simulink library "relay_housing_lib"  (Simulink 8.1)
settings: Solver=ode45  StartTime=0.0  StopTime=10.0  RelTol=1e-3
values from neighbouring files (symbols this model uses):
  F1 = xlsread('F1_relay_banshee.xlsx')    [relay_settings_init.m]
  F2 = xlsread('F2_relay_banshee.xlsx')    [relay_settings_init.m]
  F3 = xlsread('F3_relay_banshee.xlsx')    [relay_settings_init.m]
  Ts = 100E-6    (= 0.0001)    [BANSHEE_init.m]
libraries: relay_modbus_lib x42, rtio_generic_modbus x42, rtlab x3, LoadProfiles_lib x1
settings Model: Creator=re25624  LastModifiedBy=re25624

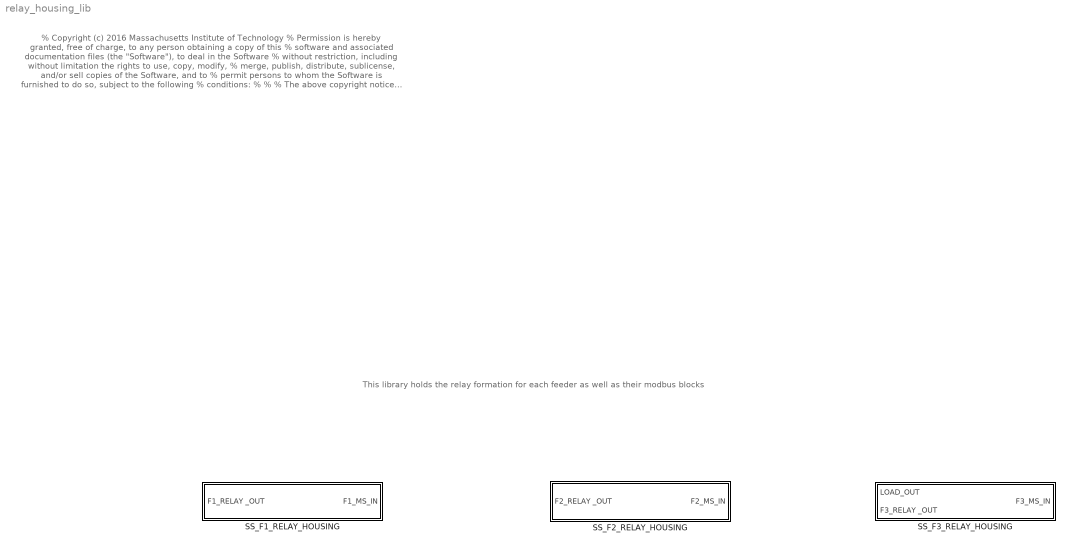
== system relay_housing_lib ==
  note: This library holds the relay formation for each feeder as well as their modbus blocks
  note: % Copyright (c) 2016 Massachusetts Institute of Technology
      | % Permission is hereby granted, free of charge, to any person obtaining a copy of this
      | % software and associated documentation files (the "Software"), to deal in the Software
      | % without restriction, including without limitation the rights to use, copy, modify,
      | % merge, publish, distribute, sublicense, and/or sell copies of the Software, and to
      | % permit persons to whom the Software is furnished to do so, subject to the following
      | % conditions:
      | %
      | %
      | % The above copyright notice and this permission notice shall be included in
      | % all copies or substantial portions of the Software.
      | %
      | % THE SOFTWARE IS PROVIDED "AS IS", WITHOUT WARRANTY OF ANY KIND, EXPRESS OR IMPLIED,
      | % INCLUDING BUT NOT LIMITED TO THE WARRANTIES OF MERCHANTABILITY, FITNESS FOR A
      | % PARTICULAR PURPOSE AND NONINFRINGEMENT. IN NO EVENT SHALL THE AUTHORS OR COPYRIGHT
      | % HOLDERS BE LIABLE FOR ANY CLAIM, DAMAGES OR OTHER LIABILITY, WHETHER IN AN ACTION
      | % OF CONTRACT, TORT OR OTHERWISE, ARISING FROM, OUT OF OR IN CONNECTION WITH THE
      | % SOFTWARE OR THE USE OR OTHER DEALINGS IN THE SOFTWARE.
      | %
      | %
      | %%
  SS_F1_RELAY_HOUSING : Subsystem
  SS_F2_RELAY_HOUSING : Subsystem
  SS_F3_RELAY_HOUSING : Subsystem

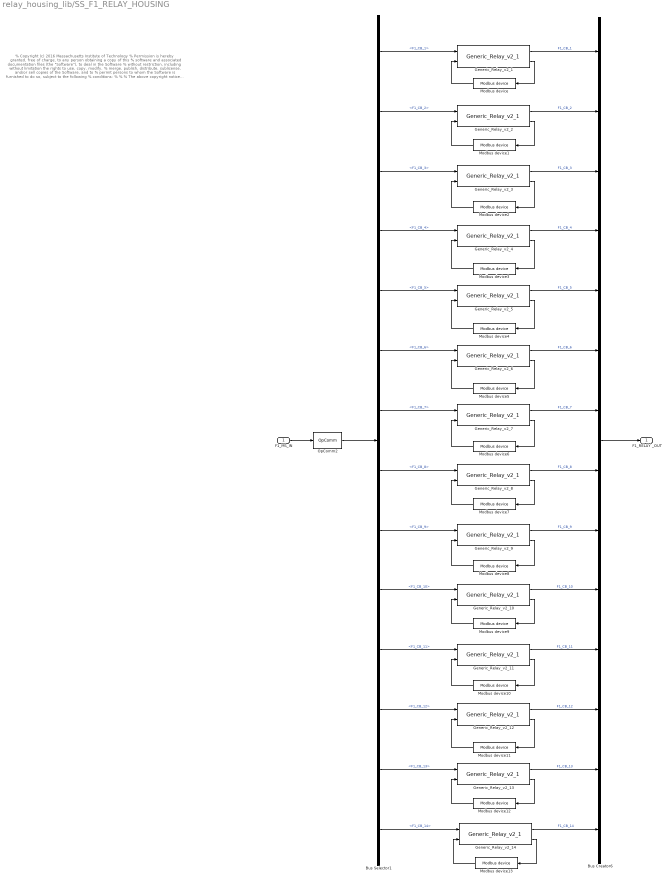
== system relay_housing_lib/SS_F1_RELAY_HOUSING ==
  note: % Copyright (c) 2016 Massachusetts Institute of Technology
      | % Permission is hereby granted, free of charge, to any person obtaining a copy of this
      | % software and associated documentation files (the "Software"), to deal in the Software
      | % without restriction, including without limitation the rights to use, copy, modify,
      | % merge, publish, distribute, sublicense, and/or sell copies of the Software, and to
      | % permit persons to whom the Software is furnished to do so, subject to the following
      | % conditions:
      | %
      | %
      | % The above copyright notice and this permission notice shall be included in
      | % all copies or substantial portions of the Software.
      | %
      | % THE SOFTWARE IS PROVIDED "AS IS", WITHOUT WARRANTY OF ANY KIND, EXPRESS OR IMPLIED,
      | % INCLUDING BUT NOT LIMITED TO THE WARRANTIES OF MERCHANTABILITY, FITNESS FOR A
      | % PARTICULAR PURPOSE AND NONINFRINGEMENT. IN NO EVENT SHALL THE AUTHORS OR COPYRIGHT
      | % HOLDERS BE LIABLE FOR ANY CLAIM, DAMAGES OR OTHER LIABILITY, WHETHER IN AN ACTION
      | % OF CONTRACT, TORT OR OTHERWISE, ARISING FROM, OUT OF OR IN CONNECTION WITH THE
      | % SOFTWARE OR THE USE OR OTHER DEALINGS IN THE SOFTWARE.
      | %
      | %
      | %%
  F1_MS_IN : Inport
  Bus Creator6 : BusCreator  Inputs=14
  Bus Selector1 : BusSelector  OutputSignals=F1_CB_1,F1_CB_2,F1_CB_3,F1_CB_4,F1_CB_5,F1_CB_6,F1_CB_7,F1_CB_8,F1_CB_9,F1_CB_10,F1_CB_11,F1_CB_12,F1_CB_13,F1_CB_14
  Generic_Relay_v2_1 : relay_modbus_lib/Generic_Relay_v2_1  Ts=Ts  relay_settings=[F1(1,:)]
  Generic_Relay_v2_10 : relay_modbus_lib/Generic_Relay_v2_1  Ts=Ts  relay_settings=[F1(10,:)]
  Generic_Relay_v2_11 : relay_modbus_lib/Generic_Relay_v2_1  Ts=Ts  relay_settings=[F1(11,:)]
  Generic_Relay_v2_12 : relay_modbus_lib/Generic_Relay_v2_1  Ts=Ts  relay_settings=[F1(12,:)]
  Generic_Relay_v2_13 : relay_modbus_lib/Generic_Relay_v2_1  Ts=Ts  relay_settings=[F1(13,:)]
  Generic_Relay_v2_14 : relay_modbus_lib/Generic_Relay_v2_1  Ts=Ts  relay_settings=[F1(14,:)]
  Generic_Relay_v2_2 : relay_modbus_lib/Generic_Relay_v2_1  Ts=Ts  relay_settings=[F1(2,:)]
  Generic_Relay_v2_3 : relay_modbus_lib/Generic_Relay_v2_1  Ts=Ts  relay_settings=[F1(3,:)]
  Generic_Relay_v2_4 : relay_modbus_lib/Generic_Relay_v2_1  Ts=Ts  relay_settings=[F1(4,:)]
  Generic_Relay_v2_5 : relay_modbus_lib/Generic_Relay_v2_1  Ts=Ts  relay_settings=[F1(5,:)]
  Generic_Relay_v2_6 : relay_modbus_lib/Generic_Relay_v2_1  Ts=Ts  relay_settings=[F1(6,:)]
  Generic_Relay_v2_7 : relay_modbus_lib/Generic_Relay_v2_1  Ts=Ts  relay_settings=[F1(7,:)]
  Generic_Relay_v2_8 : relay_modbus_lib/Generic_Relay_v2_1  Ts=Ts  relay_settings=[F1(8,:)]
  Generic_Relay_v2_9 : relay_modbus_lib/Generic_Relay_v2_1  Ts=Ts  relay_settings=[F1(9,:)]
  Modbus device : rtio_generic_modbus/Modbus device  conf_name=F1_relay_cfg1.opal  conf_name_mask=F1_relay_cfg1.xls  sample_time=Ts
  Modbus device1 : rtio_generic_modbus/Modbus device  conf_name=F1_relay_cfg2.opal  conf_name_mask=F1_relay_cfg2.xls  sample_time=Ts
  Modbus device10 : rtio_generic_modbus/Modbus device  conf_name=F1_relay_cfg11.opal  conf_name_mask=F1_relay_cfg11.xls  sample_time=Ts
  Modbus device11 : rtio_generic_modbus/Modbus device  conf_name=F1_relay_cfg12.opal  conf_name_mask=F1_relay_cfg12.xls  sample_time=Ts
  Modbus device12 : rtio_generic_modbus/Modbus device  conf_name=F1_relay_cfg13.opal  conf_name_mask=F1_relay_cfg13.xls  sample_time=Ts
  Modbus device13 : rtio_generic_modbus/Modbus device  conf_name=F1_relay_cfg14.opal  conf_name_mask=F1_relay_cfg14.xls  sample_time=Ts
  Modbus device2 : rtio_generic_modbus/Modbus device  conf_name=F1_relay_cfg3.opal  conf_name_mask=F1_relay_cfg3.xls  sample_time=Ts
  Modbus device3 : rtio_generic_modbus/Modbus device  conf_name=F1_relay_cfg4.opal  conf_name_mask=F1_relay_cfg4.xls  sample_time=Ts
  Modbus device4 : rtio_generic_modbus/Modbus device  conf_name=F1_relay_cfg5.opal  conf_name_mask=F1_relay_cfg5.xls  sample_time=Ts
  Modbus device5 : rtio_generic_modbus/Modbus device  conf_name=F1_relay_cfg6.opal  conf_name_mask=F1_relay_cfg6.xls  sample_time=Ts
  Modbus device6 : rtio_generic_modbus/Modbus device  conf_name=F1_relay_cfg7.opal  conf_name_mask=F1_relay_cfg7.xls  sample_time=Ts
  Modbus device7 : rtio_generic_modbus/Modbus device  conf_name=F1_relay_cfg8.opal  conf_name_mask=F1_relay_cfg8.xls  sample_time=Ts
  Modbus device8 : rtio_generic_modbus/Modbus device  conf_name=F1_relay_cfg9.opal  conf_name_mask=F1_relay_cfg9.xls  sample_time=Ts
  Modbus device9 : rtio_generic_modbus/Modbus device  conf_name=F1_relay_cfg10.opal  conf_name_mask=F1_relay_cfg10.xls  sample_time=Ts
  OpComm2 : rtlab/OpComm  nbport=1  groupe_acq=1  subsys_rate=0  st=0  Synchronization=on  Interpolation=on  Threshold=1.0  Missed_Data=off  Sim_Time=off  Samples=off  dynSigOut=off  from_console=0  warning_done=off  writeOpCommFile=off  Offset=off
  F1_RELAY _OUT : Outport
  wires:
  Bus Selector1/14 -> Generic_Relay_v2_14/1  "<F1_CB_14>"
  Generic_Relay_v2_14/1 -> Bus Creator6/14  "F1_CB_14"
  Generic_Relay_v2_14/2 -> Modbus device13/1
  Modbus device13/1 -> Generic_Relay_v2_14/2
  Generic_Relay_v2_3/1 -> Bus Creator6/3  "F1_CB_3"
  Generic_Relay_v2_4/1 -> Bus Creator6/4  "F1_CB_4"
  Generic_Relay_v2_5/1 -> Bus Creator6/5  "F1_CB_5"
  Generic_Relay_v2_6/1 -> Bus Creator6/6  "F1_CB_6"
  Generic_Relay_v2_7/1 -> Bus Creator6/7  "F1_CB_7"
  Generic_Relay_v2_8/1 -> Bus Creator6/8  "F1_CB_8"
  Generic_Relay_v2_9/1 -> Bus Creator6/9  "F1_CB_9"
  Generic_Relay_v2_10/1 -> Bus Creator6/10  "F1_CB_10"
  Generic_Relay_v2_11/1 -> Bus Creator6/11  "F1_CB_11"
  Generic_Relay_v2_12/1 -> Bus Creator6/12  "F1_CB_12"
  Generic_Relay_v2_13/1 -> Bus Creator6/13  "F1_CB_13"
  Bus Selector1/13 -> Generic_Relay_v2_13/1  "<F1_CB_13>"
  Bus Selector1/12 -> Generic_Relay_v2_12/1  "<F1_CB_12>"
  Bus Selector1/11 -> Generic_Relay_v2_11/1  "<F1_CB_11>"
  Bus Selector1/10 -> Generic_Relay_v2_10/1  "<F1_CB_10>"
  Bus Selector1/9 -> Generic_Relay_v2_9/1  "<F1_CB_9>"
  Bus Selector1/8 -> Generic_Relay_v2_8/1  "<F1_CB_8>"
  Bus Selector1/7 -> Generic_Relay_v2_7/1  "<F1_CB_7>"
  Bus Selector1/6 -> Generic_Relay_v2_6/1  "<F1_CB_6>"
  Bus Selector1/5 -> Generic_Relay_v2_5/1  "<F1_CB_5>"
  Bus Selector1/4 -> Generic_Relay_v2_4/1  "<F1_CB_4>"
  Bus Selector1/3 -> Generic_Relay_v2_3/1  "<F1_CB_3>"
  Generic_Relay_v2_2/1 -> Bus Creator6/2  "F1_CB_2"
  Bus Selector1/2 -> Generic_Relay_v2_2/1  "<F1_CB_2>"
  Bus Creator6/1 -> F1_RELAY _OUT/1
  Generic_Relay_v2_1/1 -> Bus Creator6/1  "F1_CB_1"
  Bus Selector1/1 -> Generic_Relay_v2_1/1  "<F1_CB_1>"
  F1_MS_IN/1 -> OpComm2/1
  Modbus device/1 -> Generic_Relay_v2_1/2
  Generic_Relay_v2_1/2 -> Modbus device/1
  Modbus device1/1 -> Generic_Relay_v2_2/2
  Generic_Relay_v2_2/2 -> Modbus device1/1
  Generic_Relay_v2_3/2 -> Modbus device2/1
  Modbus device2/1 -> Generic_Relay_v2_3/2
  Generic_Relay_v2_4/2 -> Modbus device3/1
  Modbus device3/1 -> Generic_Relay_v2_4/2
  Generic_Relay_v2_5/2 -> Modbus device4/1
  Modbus device4/1 -> Generic_Relay_v2_5/2
  Generic_Relay_v2_6/2 -> Modbus device5/1
  Modbus device5/1 -> Generic_Relay_v2_6/2
  Generic_Relay_v2_7/2 -> Modbus device6/1
  Modbus device6/1 -> Generic_Relay_v2_7/2
  Generic_Relay_v2_8/2 -> Modbus device7/1
  Modbus device7/1 -> Generic_Relay_v2_8/2
  Generic_Relay_v2_9/2 -> Modbus device8/1
  Modbus device8/1 -> Generic_Relay_v2_9/2
  Generic_Relay_v2_10/2 -> Modbus device9/1
  Modbus device9/1 -> Generic_Relay_v2_10/2
  Generic_Relay_v2_11/2 -> Modbus device10/1
  Modbus device10/1 -> Generic_Relay_v2_11/2
  Generic_Relay_v2_12/2 -> Modbus device11/1
  Modbus device11/1 -> Generic_Relay_v2_12/2
  Generic_Relay_v2_13/2 -> Modbus device12/1
  Modbus device12/1 -> Generic_Relay_v2_13/2
  OpComm2/1 -> Bus Selector1/1

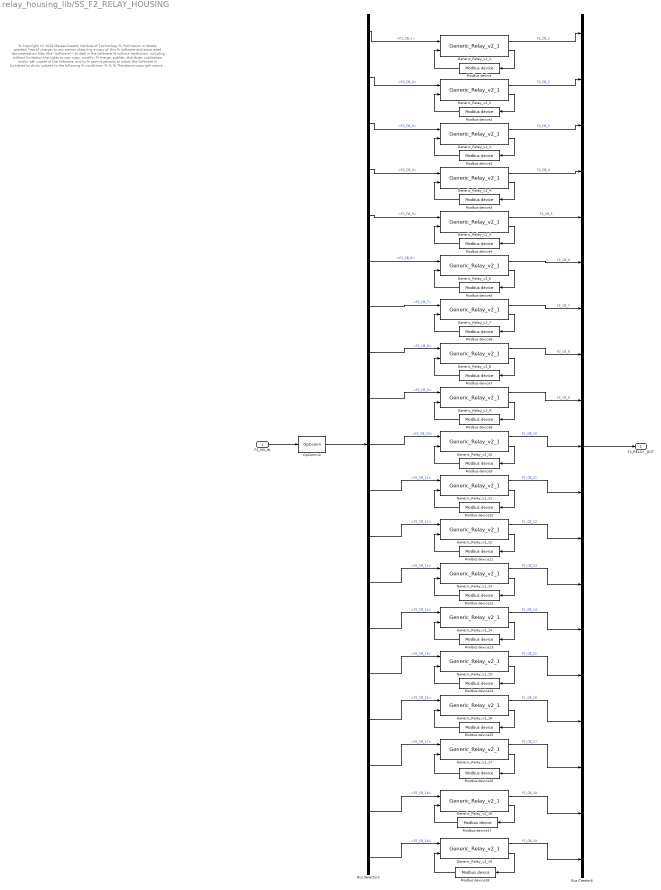
== system relay_housing_lib/SS_F2_RELAY_HOUSING ==
  note: % Copyright (c) 2016 Massachusetts Institute of Technology
      | % Permission is hereby granted, free of charge, to any person obtaining a copy of this
      | % software and associated documentation files (the "Software"), to deal in the Software
      | % without restriction, including without limitation the rights to use, copy, modify,
      | % merge, publish, distribute, sublicense, and/or sell copies of the Software, and to
      | % permit persons to whom the Software is furnished to do so, subject to the following
      | % conditions:
      | %
      | %
      | % The above copyright notice and this permission notice shall be included in
      | % all copies or substantial portions of the Software.
      | %
      | % THE SOFTWARE IS PROVIDED "AS IS", WITHOUT WARRANTY OF ANY KIND, EXPRESS OR IMPLIED,
      | % INCLUDING BUT NOT LIMITED TO THE WARRANTIES OF MERCHANTABILITY, FITNESS FOR A
      | % PARTICULAR PURPOSE AND NONINFRINGEMENT. IN NO EVENT SHALL THE AUTHORS OR COPYRIGHT
      | % HOLDERS BE LIABLE FOR ANY CLAIM, DAMAGES OR OTHER LIABILITY, WHETHER IN AN ACTION
      | % OF CONTRACT, TORT OR OTHERWISE, ARISING FROM, OUT OF OR IN CONNECTION WITH THE
      | % SOFTWARE OR THE USE OR OTHER DEALINGS IN THE SOFTWARE.
      | %
      | %
      | %%
  F2_MS_IN : Inport
  Bus Creator6 : BusCreator  Inputs=19
  Bus Selector2 : BusSelector  OutputSignals=F2_CB_1,F2_CB_2,F2_CB_3,F2_CB_4,F2_CB_5,F2_CB_6,F2_CB_7,F2_CB_8,F2_CB_9,F2_CB_10,F2_CB_11,F2_CB_12,F2_CB_13,F2_CB_14,F2_CB_15,F2_CB_16,F2_CB_17,F2_CB_18,F2_CB_19
  Generic_Relay_v2_1 : relay_modbus_lib/Generic_Relay_v2_1  Ts=Ts  relay_settings=[F2(1,:)]
  Generic_Relay_v2_10 : relay_modbus_lib/Generic_Relay_v2_1  Ts=Ts  relay_settings=[F2(10,:)]
  Generic_Relay_v2_11 : relay_modbus_lib/Generic_Relay_v2_1  Ts=Ts  relay_settings=[F2(11,:)]
  Generic_Relay_v2_12 : relay_modbus_lib/Generic_Relay_v2_1  Ts=Ts  relay_settings=[F2(12,:)]
  Generic_Relay_v2_13 : relay_modbus_lib/Generic_Relay_v2_1  Ts=Ts  relay_settings=[F2(13,:)]
  Generic_Relay_v2_14 : relay_modbus_lib/Generic_Relay_v2_1  Ts=Ts  relay_settings=[F2(14,:)]
  Generic_Relay_v2_15 : relay_modbus_lib/Generic_Relay_v2_1  Ts=Ts  relay_settings=[F2(15,:)]
  Generic_Relay_v2_16 : relay_modbus_lib/Generic_Relay_v2_1  Ts=Ts  relay_settings=[F2(16,:)]
  Generic_Relay_v2_17 : relay_modbus_lib/Generic_Relay_v2_1  Ts=Ts  relay_settings=[F2(17,:)]
  Generic_Relay_v2_18 : relay_modbus_lib/Generic_Relay_v2_1  Ts=Ts  relay_settings=[F2(18,:)]
  Generic_Relay_v2_19 : relay_modbus_lib/Generic_Relay_v2_1  Ts=Ts  relay_settings=[F2(19,:)]
  Generic_Relay_v2_2 : relay_modbus_lib/Generic_Relay_v2_1  Ts=Ts  relay_settings=[F2(2,:)]
  Generic_Relay_v2_3 : relay_modbus_lib/Generic_Relay_v2_1  Ts=Ts  relay_settings=[F2(3,:)]
  Generic_Relay_v2_4 : relay_modbus_lib/Generic_Relay_v2_1  Ts=Ts  relay_settings=[F2(4,:)]
  Generic_Relay_v2_5 : relay_modbus_lib/Generic_Relay_v2_1  Ts=Ts  relay_settings=[F2(5,:)]
  Generic_Relay_v2_6 : relay_modbus_lib/Generic_Relay_v2_1  Ts=Ts  relay_settings=[F2(6,:)]
  Generic_Relay_v2_7 : relay_modbus_lib/Generic_Relay_v2_1  Ts=Ts  relay_settings=[F2(7,:)]
  Generic_Relay_v2_8 : relay_modbus_lib/Generic_Relay_v2_1  Ts=Ts  relay_settings=[F2(8,:)]
  Generic_Relay_v2_9 : relay_modbus_lib/Generic_Relay_v2_1  Ts=Ts  relay_settings=[F2(9,:)]
  Modbus device : rtio_generic_modbus/Modbus device  conf_name=F2_relay_cfg1.opal  conf_name_mask=F2_relay_cfg1.xls  sample_time=Ts
  Modbus device1 : rtio_generic_modbus/Modbus device  conf_name=F2_relay_cfg2.opal  conf_name_mask=F2_relay_cfg2.xls  sample_time=Ts
  Modbus device10 : rtio_generic_modbus/Modbus device  conf_name=F2_relay_cfg11.opal  conf_name_mask=F2_relay_cfg11.xls  sample_time=Ts
  Modbus device11 : rtio_generic_modbus/Modbus device  conf_name=F2_relay_cfg12.opal  conf_name_mask=F2_relay_cfg12.xls  sample_time=Ts
  Modbus device12 : rtio_generic_modbus/Modbus device  conf_name=F2_relay_cfg13.opal  conf_name_mask=F2_relay_cfg13.xls  sample_time=Ts
  Modbus device13 : rtio_generic_modbus/Modbus device  conf_name=F2_relay_cfg14.opal  conf_name_mask=F2_relay_cfg14.xls  sample_time=Ts
  Modbus device14 : rtio_generic_modbus/Modbus device  conf_name=F2_relay_cfg15.opal  conf_name_mask=F2_relay_cfg15.xls  sample_time=Ts
  Modbus device15 : rtio_generic_modbus/Modbus device  conf_name=F2_relay_cfg16.opal  conf_name_mask=F2_relay_cfg16.xls  sample_time=Ts
  Modbus device16 : rtio_generic_modbus/Modbus device  conf_name=F2_relay_cfg17.opal  conf_name_mask=F2_relay_cfg17.xls  sample_time=Ts
  Modbus device17 : rtio_generic_modbus/Modbus device  conf_name=F2_relay_cfg18.opal  conf_name_mask=F2_relay_cfg18.xls  sample_time=Ts
  Modbus device18 : rtio_generic_modbus/Modbus device  conf_name=F2_relay_cfg19.opal  conf_name_mask=F2_relay_cfg19.xls  sample_time=Ts
  Modbus device2 : rtio_generic_modbus/Modbus device  conf_name=F2_relay_cfg3.opal  conf_name_mask=F2_relay_cfg3.xls  sample_time=Ts
  Modbus device3 : rtio_generic_modbus/Modbus device  conf_name=F2_relay_cfg4.opal  conf_name_mask=F2_relay_cfg4.xls  sample_time=Ts
  Modbus device4 : rtio_generic_modbus/Modbus device  conf_name=F2_relay_cfg5.opal  conf_name_mask=F2_relay_cfg5.xls  sample_time=Ts
  Modbus device5 : rtio_generic_modbus/Modbus device  conf_name=F2_relay_cfg6.opal  conf_name_mask=F2_relay_cfg6.xls  sample_time=Ts
  Modbus device6 : rtio_generic_modbus/Modbus device  conf_name=F2_relay_cfg7.opal  conf_name_mask=F2_relay_cfg7.xls  sample_time=Ts
  Modbus device7 : rtio_generic_modbus/Modbus device  conf_name=F2_relay_cfg8.opal  conf_name_mask=F2_relay_cfg8.xls  sample_time=Ts
  Modbus device8 : rtio_generic_modbus/Modbus device  conf_name=F2_relay_cfg9.opal  conf_name_mask=F2_relay_cfg9.xls  sample_time=Ts
  Modbus device9 : rtio_generic_modbus/Modbus device  conf_name=F2_relay_cfg10.opal  conf_name_mask=F2_relay_cfg10.xls  sample_time=Ts
  OpComm2 : rtlab/OpComm  nbport=1  groupe_acq=1  subsys_rate=0  st=0  Synchronization=on  Interpolation=on  Threshold=1.0  Missed_Data=off  Sim_Time=off  Samples=off  dynSigOut=off  from_console=0  warning_done=off  writeOpCommFile=off  Offset=off
  F2_RELAY _OUT : Outport
  wires:
  Bus Selector2/18 -> Generic_Relay_v2_18/1  "<F2_CB_18>"
  Bus Selector2/19 -> Generic_Relay_v2_19/1  "<F2_CB_19>"
  Generic_Relay_v2_19/1 -> Bus Creator6/19  "F2_CB_19"
  Generic_Relay_v2_18/1 -> Bus Creator6/18  "F2_CB_18"
  Generic_Relay_v2_18/2 -> Modbus device17/1
  Modbus device17/1 -> Generic_Relay_v2_18/2
  Generic_Relay_v2_19/2 -> Modbus device18/1
  Modbus device18/1 -> Generic_Relay_v2_19/2
  Bus Selector2/17 -> Generic_Relay_v2_17/1  "<F2_CB_17>"
  Generic_Relay_v2_17/1 -> Bus Creator6/17  "F2_CB_17"
  Generic_Relay_v2_6/1 -> Bus Creator6/6  "F2_CB_6"
  Generic_Relay_v2_5/1 -> Bus Creator6/5  "F2_CB_5"
  Generic_Relay_v2_4/1 -> Bus Creator6/4  "F2_CB_4"
  Generic_Relay_v2_3/1 -> Bus Creator6/3  "F2_CB_3"
  Generic_Relay_v2_2/1 -> Bus Creator6/2  "F2_CB_2"
  Generic_Relay_v2_7/1 -> Bus Creator6/7  "F2_CB_7"
  Generic_Relay_v2_8/1 -> Bus Creator6/8  "F2_CB_8"
  Generic_Relay_v2_9/1 -> Bus Creator6/9  "F2_CB_9"
  Generic_Relay_v2_10/1 -> Bus Creator6/10  "F2_CB_10"
  Generic_Relay_v2_11/1 -> Bus Creator6/11  "F2_CB_11"
  Generic_Relay_v2_16/1 -> Bus Creator6/16  "F2_CB_16"
  Generic_Relay_v2_15/1 -> Bus Creator6/15  "F2_CB_15"
  Generic_Relay_v2_14/1 -> Bus Creator6/14  "F2_CB_14"
  Generic_Relay_v2_13/1 -> Bus Creator6/13  "F2_CB_13"
  Generic_Relay_v2_12/1 -> Bus Creator6/12  "F2_CB_12"
  Bus Selector2/16 -> Generic_Relay_v2_16/1  "<F2_CB_16>"
  Bus Selector2/15 -> Generic_Relay_v2_15/1  "<F2_CB_15>"
  Bus Selector2/14 -> Generic_Relay_v2_14/1  "<F2_CB_14>"
  Bus Selector2/13 -> Generic_Relay_v2_13/1  "<F2_CB_13>"
  Bus Selector2/12 -> Generic_Relay_v2_12/1  "<F2_CB_12>"
  Bus Selector2/11 -> Generic_Relay_v2_11/1  "<F2_CB_11>"
  Bus Selector2/10 -> Generic_Relay_v2_10/1  "<F2_CB_10>"
  Bus Selector2/9 -> Generic_Relay_v2_9/1  "<F2_CB_9>"
  Bus Selector2/8 -> Generic_Relay_v2_8/1  "<F2_CB_8>"
  Bus Selector2/7 -> Generic_Relay_v2_7/1  "<F2_CB_7>"
  Bus Selector2/6 -> Generic_Relay_v2_6/1  "<F2_CB_6>"
  Bus Selector2/5 -> Generic_Relay_v2_5/1  "<F2_CB_5>"
  Bus Selector2/4 -> Generic_Relay_v2_4/1  "<F2_CB_4>"
  Bus Selector2/3 -> Generic_Relay_v2_3/1  "<F2_CB_3>"
  Bus Selector2/2 -> Generic_Relay_v2_2/1  "<F2_CB_2>"
  Generic_Relay_v2_1/1 -> Bus Creator6/1  "F2_CB_1"
  Bus Selector2/1 -> Generic_Relay_v2_1/1  "<F2_CB_1>"
  F2_MS_IN/1 -> OpComm2/1
  Bus Creator6/1 -> F2_RELAY _OUT/1
  Generic_Relay_v2_1/2 -> Modbus device/1
  Modbus device/1 -> Generic_Relay_v2_1/2
  Generic_Relay_v2_2/2 -> Modbus device1/1
  Modbus device1/1 -> Generic_Relay_v2_2/2
  Generic_Relay_v2_3/2 -> Modbus device2/1
  Modbus device2/1 -> Generic_Relay_v2_3/2
  Generic_Relay_v2_4/2 -> Modbus device3/1
  Modbus device3/1 -> Generic_Relay_v2_4/2
  Generic_Relay_v2_5/2 -> Modbus device4/1
  Modbus device4/1 -> Generic_Relay_v2_5/2
  Modbus device5/1 -> Generic_Relay_v2_6/2
  Generic_Relay_v2_6/2 -> Modbus device5/1
  Generic_Relay_v2_7/2 -> Modbus device6/1
  Modbus device6/1 -> Generic_Relay_v2_7/2
  Generic_Relay_v2_8/2 -> Modbus device7/1
  Modbus device7/1 -> Generic_Relay_v2_8/2
  Generic_Relay_v2_9/2 -> Modbus device8/1
  Modbus device8/1 -> Generic_Relay_v2_9/2
  Generic_Relay_v2_10/2 -> Modbus device9/1
  Modbus device9/1 -> Generic_Relay_v2_10/2
  Generic_Relay_v2_11/2 -> Modbus device10/1
  Modbus device10/1 -> Generic_Relay_v2_11/2
  Generic_Relay_v2_12/2 -> Modbus device11/1
  Modbus device11/1 -> Generic_Relay_v2_12/2
  Modbus device12/1 -> Generic_Relay_v2_13/2
  Generic_Relay_v2_13/2 -> Modbus device12/1
  Generic_Relay_v2_14/2 -> Modbus device13/1
  Modbus device13/1 -> Generic_Relay_v2_14/2
  Generic_Relay_v2_15/2 -> Modbus device14/1
  Modbus device14/1 -> Generic_Relay_v2_15/2
  Generic_Relay_v2_16/2 -> Modbus device15/1
  Modbus device15/1 -> Generic_Relay_v2_16/2
  Generic_Relay_v2_17/2 -> Modbus device16/1
  Modbus device16/1 -> Generic_Relay_v2_17/2
  OpComm2/1 -> Bus Selector2/1

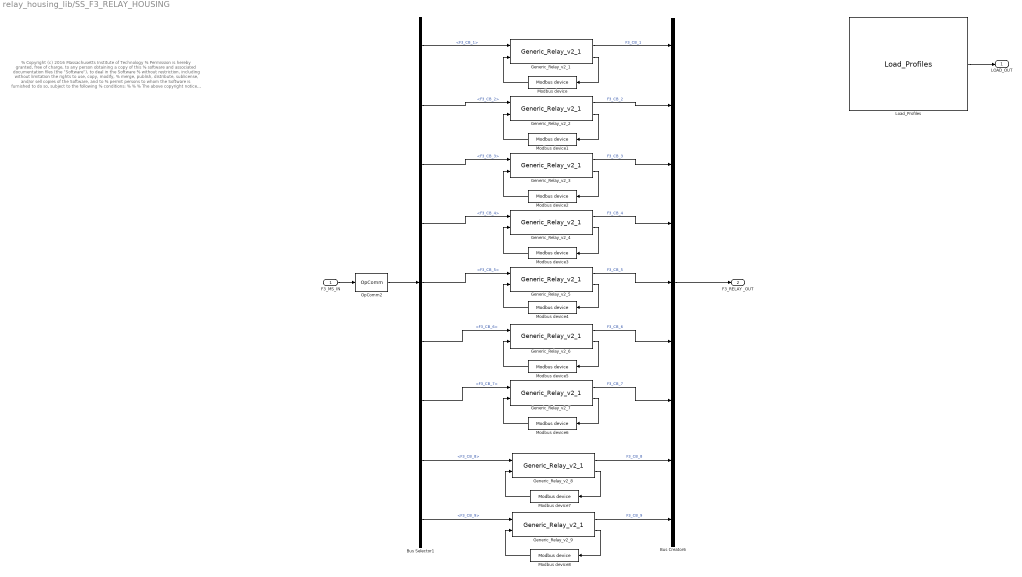
== system relay_housing_lib/SS_F3_RELAY_HOUSING ==
  note: % Copyright (c) 2016 Massachusetts Institute of Technology
      | % Permission is hereby granted, free of charge, to any person obtaining a copy of this
      | % software and associated documentation files (the "Software"), to deal in the Software
      | % without restriction, including without limitation the rights to use, copy, modify,
      | % merge, publish, distribute, sublicense, and/or sell copies of the Software, and to
      | % permit persons to whom the Software is furnished to do so, subject to the following
      | % conditions:
      | %
      | %
      | % The above copyright notice and this permission notice shall be included in
      | % all copies or substantial portions of the Software.
      | %
      | % THE SOFTWARE IS PROVIDED "AS IS", WITHOUT WARRANTY OF ANY KIND, EXPRESS OR IMPLIED,
      | % INCLUDING BUT NOT LIMITED TO THE WARRANTIES OF MERCHANTABILITY, FITNESS FOR A
      | % PARTICULAR PURPOSE AND NONINFRINGEMENT. IN NO EVENT SHALL THE AUTHORS OR COPYRIGHT
      | % HOLDERS BE LIABLE FOR ANY CLAIM, DAMAGES OR OTHER LIABILITY, WHETHER IN AN ACTION
      | % OF CONTRACT, TORT OR OTHERWISE, ARISING FROM, OUT OF OR IN CONNECTION WITH THE
      | % SOFTWARE OR THE USE OR OTHER DEALINGS IN THE SOFTWARE.
      | %
      | %
      | %%
  F3_MS_IN : Inport
  Bus Creator6 : BusCreator  Inputs=9
  Bus Selector1 : BusSelector  OutputSignals=F3_CB_1,F3_CB_2,F3_CB_3,F3_CB_4,F3_CB_5,F3_CB_6,F3_CB_7,F3_CB_8,F3_CB_9
  Generic_Relay_v2_1 : relay_modbus_lib/Generic_Relay_v2_1  Ts=Ts  relay_settings=[F3(1,:)]
  Generic_Relay_v2_2 : relay_modbus_lib/Generic_Relay_v2_1  Ts=Ts  relay_settings=[F3(2,:)]
  Generic_Relay_v2_3 : relay_modbus_lib/Generic_Relay_v2_1  Ts=Ts  relay_settings=[F3(3,:)]
  Generic_Relay_v2_4 : relay_modbus_lib/Generic_Relay_v2_1  Ts=Ts  relay_settings=[F3(4,:)]
  Generic_Relay_v2_5 : relay_modbus_lib/Generic_Relay_v2_1  Ts=Ts  relay_settings=[F3(5,:)]
  Generic_Relay_v2_6 : relay_modbus_lib/Generic_Relay_v2_1  Ts=Ts  relay_settings=[F3(6,:)]
  Generic_Relay_v2_7 : relay_modbus_lib/Generic_Relay_v2_1  Ts=Ts  relay_settings=[F3(7,:)]
  Generic_Relay_v2_8 : relay_modbus_lib/Generic_Relay_v2_1  Ts=Ts  relay_settings=[F3(8,:)]
  Generic_Relay_v2_9 : relay_modbus_lib/Generic_Relay_v2_1  Ts=Ts  relay_settings=[F3(9,:)]
  Load_Profiles : LoadProfiles_lib/Load_Profiles
  Modbus device : rtio_generic_modbus/Modbus device  conf_name=F3_relay_cfg1.opal  conf_name_mask=F3_relay_cfg1.xls  sample_time=Ts
  Modbus device1 : rtio_generic_modbus/Modbus device  conf_name=F3_relay_cfg2.opal  conf_name_mask=F3_relay_cfg2.xls  sample_time=Ts
  Modbus device2 : rtio_generic_modbus/Modbus device  conf_name=F3_relay_cfg3.opal  conf_name_mask=F3_relay_cfg3.xls  sample_time=Ts
  Modbus device3 : rtio_generic_modbus/Modbus device  conf_name=F3_relay_cfg4.opal  conf_name_mask=F3_relay_cfg4.xls  sample_time=Ts
  Modbus device4 : rtio_generic_modbus/Modbus device  conf_name=F3_relay_cfg5.opal  conf_name_mask=F3_relay_cfg5.xls  sample_time=Ts
  Modbus device5 : rtio_generic_modbus/Modbus device  conf_name=F3_relay_cfg6.opal  conf_name_mask=F3_relay_cfg6.xls  sample_time=Ts
  Modbus device6 : rtio_generic_modbus/Modbus device  conf_name=F3_relay_cfg7.opal  conf_name_mask=F3_relay_cfg7.xls  sample_time=Ts
  Modbus device7 : rtio_generic_modbus/Modbus device  conf_name=F3_relay_cfg8.opal  conf_name_mask=F3_relay_cfg8.xls  sample_time=Ts
  Modbus device8 : rtio_generic_modbus/Modbus device  conf_name=F3_relay_cfg9.opal  conf_name_mask=F3_relay_cfg9.xls  sample_time=Ts
  OpComm2 : rtlab/OpComm  nbport=1  groupe_acq=1  subsys_rate=0  st=0  Synchronization=on  Interpolation=on  Threshold=1.0  Missed_Data=off  Sim_Time=off  Samples=off  dynSigOut=off  from_console=0  warning_done=off  writeOpCommFile=off  Offset=off
  LOAD_OUT : Outport
  F3_RELAY _OUT : Outport  Port=2
  wires:
  Bus Selector1/8 -> Generic_Relay_v2_8/1  "<F3_CB_8>"
  Bus Selector1/9 -> Generic_Relay_v2_9/1  "<F3_CB_9>"
  Generic_Relay_v2_9/1 -> Bus Creator6/9  "F3_CB_9"
  Generic_Relay_v2_8/1 -> Bus Creator6/8  "F3_CB_8"
  Modbus device8/1 -> Generic_Relay_v2_9/2
  Generic_Relay_v2_9/2 -> Modbus device8/1
  Generic_Relay_v2_8/2 -> Modbus device7/1
  Modbus device7/1 -> Generic_Relay_v2_8/2
  Bus Creator6/1 -> F3_RELAY _OUT/1
  Generic_Relay_v2_7/1 -> Bus Creator6/7  "F3_CB_7"
  Generic_Relay_v2_6/1 -> Bus Creator6/6  "F3_CB_6"
  Generic_Relay_v2_5/1 -> Bus Creator6/5  "F3_CB_5"
  Generic_Relay_v2_4/1 -> Bus Creator6/4  "F3_CB_4"
  Generic_Relay_v2_3/1 -> Bus Creator6/3  "F3_CB_3"
  Generic_Relay_v2_2/1 -> Bus Creator6/2  "F3_CB_2"
  Generic_Relay_v2_1/1 -> Bus Creator6/1  "F3_CB_1"
  Bus Selector1/7 -> Generic_Relay_v2_7/1  "<F3_CB_7>"
  Bus Selector1/6 -> Generic_Relay_v2_6/1  "<F3_CB_6>"
  Bus Selector1/5 -> Generic_Relay_v2_5/1  "<F3_CB_5>"
  Bus Selector1/4 -> Generic_Relay_v2_4/1  "<F3_CB_4>"
  Bus Selector1/3 -> Generic_Relay_v2_3/1  "<F3_CB_3>"
  Bus Selector1/2 -> Generic_Relay_v2_2/1  "<F3_CB_2>"
  Bus Selector1/1 -> Generic_Relay_v2_1/1  "<F3_CB_1>"
  F3_MS_IN/1 -> OpComm2/1
  Modbus device6/1 -> Generic_Relay_v2_7/2
  Generic_Relay_v2_7/2 -> Modbus device6/1
  Generic_Relay_v2_6/2 -> Modbus device5/1
  Modbus device5/1 -> Generic_Relay_v2_6/2
  Modbus device4/1 -> Generic_Relay_v2_5/2
  Generic_Relay_v2_5/2 -> Modbus device4/1
  Modbus device3/1 -> Generic_Relay_v2_4/2
  Generic_Relay_v2_4/2 -> Modbus device3/1
  Generic_Relay_v2_3/2 -> Modbus device2/1
  Modbus device2/1 -> Generic_Relay_v2_3/2
  Modbus device1/1 -> Generic_Relay_v2_2/2
  Generic_Relay_v2_2/2 -> Modbus device1/1
  Modbus device/1 -> Generic_Relay_v2_1/2
  Generic_Relay_v2_1/2 -> Modbus device/1
  OpComm2/1 -> Bus Selector1/1
  Load_Profiles/1 -> LOAD_OUT/1
